simulink model "thyristor_3phase_common_point"  (R2015a)
settings: Solver=ode45  StartTime=0.0  StopTime=0.03  MaxStep=1/10000  RelTol=1e-3
libraries: powerlib x10, simulink x3
settings Model: Creator=Windows 10  LastModifiedBy=Windows 10

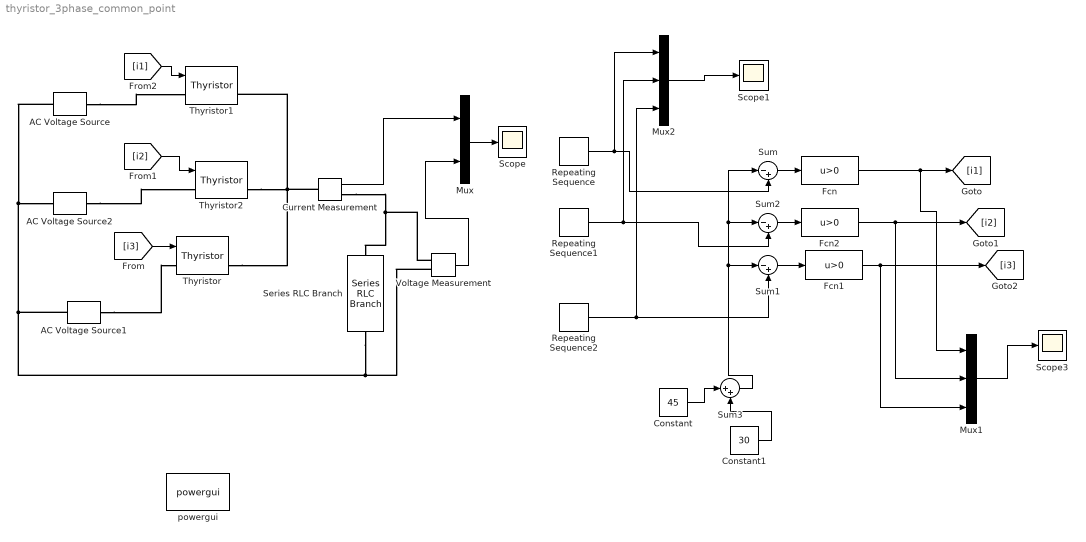
== system thyristor_3phase_common_point ==
  AC Voltage Source : powerlib/Electrical Sources/AC Voltage Source  Amplitude=300  Phase=0  Frequency=50  SampleTime=0  Measurements=None
  AC Voltage Source1 : powerlib/Electrical Sources/AC Voltage Source  Amplitude=300  Phase=120  Frequency=50  SampleTime=0  Measurements=None
  AC Voltage Source2 : powerlib/Electrical Sources/AC Voltage Source  Amplitude=300  Phase=-120  Frequency=50  SampleTime=0  Measurements=None
  Constant : Constant  Value=45
  Constant1 : Constant  Value=30
  Current Measurement : powerlib/Measurements/Current Measurement  PhasorSimulation=off  OutputType=Complex  PSBequivalent=0
  Fcn : Fcn  Expr=u>0
  Fcn1 : Fcn  Expr=u>0
  Fcn2 : Fcn  Expr=u>0
  Mux : Mux  Inputs=2
  Mux1 : Mux  Inputs=3
  Mux2 : Mux  Inputs=3
  Repeating Sequence : simulink/Sources/Repeating Sequence  rep_seq_t=[0 10 10.0001 20]*1e-3  rep_seq_y=[0 180 -180 0]
  Repeating Sequence1 : simulink/Sources/Repeating Sequence  rep_seq_t=[0 5*20/6 (5*20/6+0.0010) 20]*1e-3  rep_seq_y=[-120 180 -180 -120]
  Repeating Sequence2 : simulink/Sources/Repeating Sequence  rep_seq_t=[0 20/6 20/6+0.001 20]*1e-3  rep_seq_y=[120 180 -180 120]
  Scope : Scope
  Scope1 : Scope
  Scope3 : Scope
      settings: SaveName=ScopeData3
  Series RLC Branch : powerlib/Elements/Series RLC Branch  LConnTagsString=__new0  RConnTagsString=__new0  BranchType=R  Resistance=2  Inductance=1e-3  SetiL0=off  InitialCurrent=0  Capacitance=1e-6  Setx0=off  InitialVoltage=0  Measurements=None
  Sum : Sum  Inputs=|-+
  Sum1 : Sum  Inputs=|-+
  Sum2 : Sum  Inputs=|-+
  Sum3 : Sum  Inputs=|++
  Thyristor : powerlib/Power Electronics/Thyristor  Ron=0.001  Lon=0  Vf=0.8  IC=0  Rs=500  Cs=250e-9  Measurements=on
  Thyristor1 : powerlib/Power Electronics/Thyristor  Ron=0.001  Lon=0  Vf=0.8  IC=0  Rs=500  Cs=250e-9  Measurements=on
  Thyristor2 : powerlib/Power Electronics/Thyristor  Ron=0.001  Lon=0  Vf=0.8  IC=0  Rs=500  Cs=250e-9  Measurements=on
  Voltage Measurement : powerlib/Measurements/Voltage Measurement  PhasorSimulation=off  OutputType=Complex  PSBequivalent=0
  powergui : powerlib/powergui  Priority=1  SimulationMode=Continuous  SolverType=Tustin/Backward Euler (TBE)  SampleTime=50e-6  frequency=60  SPID=off  DisableSnubberDevices=off  DisableRonSwitches=off  DisableVfSwitches=off  SwTol=0  DisplayEquations=off  Interpol=off  methode=off  Ts=100  FunctionMessages=off  echomessages=off  HookPort=off  EnableUseOfTLC=off  x0status=blocks  frequencyindice=50  Pbase=100e6  ErrMax=1e-4  Iterations=50  UnitsV=kV  UnitsW=MW  buscounter=0  RestoreLinks=warning  ResistiveCurrentMeasurement=off  Frange=[0:2:500]  Ylog=off  Xlog=on  ShowGrid=off  save=off  variable=ZData  structure=0  ZoomFFT=off  StartTime=0.0  cycles=1  DisplayStyle=1  fundamental=60  FreqAxis=off  MaxFrequency=1000  frequencyindicesteady=1  RmsSteady=1  display=off
  wires:
  Voltage Measurement/1 -> Mux/2
  Current Measurement/1 -> Mux/1
  Mux/1 -> Scope/1
  Repeating Sequence/1 -> Sum/2, Mux2/1
  Repeating Sequence1/1 -> Sum2/2, Mux2/2
  Repeating Sequence2/1 -> Sum1/2, Mux2/3
  Constant/1 -> Sum3/1
  Constant1/1 -> Sum3/2
  Sum3/1 -> Sum1/1, Sum2/1, Sum/1
  Sum2/1 -> Fcn2/1
  Sum1/1 -> Fcn1/1
  Sum/1 -> Fcn/1
  Mux2/1 -> Scope1/1
  Mux1/1 -> Scope3/1
  [i2] -> Thyristor2/1
  [i3] -> Thyristor/1
  [i1] -> Thyristor1/1
  Fcn2/1 -> Mux1/2, [i2]
  Fcn1/1 -> Mux1/3, [i3]
  Fcn/1 -> Mux1/1, [i1]
  connections:
  AC Voltage Source/LConn1 -- Voltage Measurement/LConn2 -- Series RLC Branch/RConn1 -- AC Voltage Source1/LConn1 -- AC Voltage Source2/LConn1
  AC Voltage Source/RConn1 -- Thyristor1/LConn1
  AC Voltage Source2/RConn1 -- Thyristor2/LConn1
  AC Voltage Source1/RConn1 -- Thyristor/LConn1
  Thyristor2/RConn1 -- Thyristor/RConn1 -- Current Measurement/LConn1 -- Thyristor1/RConn1
  Current Measurement/RConn1 -- Voltage Measurement/LConn1 -- Series RLC Branch/LConn1
